simulink model "Exp_300_MPCLinearization"  (R2016a)
settings: Solver=ode45  StartTime=0.0  StopTime=700  RelTol=1e-3
StartFcn:
  | clear all
libraries: mpclib x1
settings Model: Creator=johnh  LastModifiedBy=tiago
settings DataIOCC: SaveFormat=StructureWithTime
settings HardwareCC: ProdWordSize=32  ProdHWDeviceType=Specified
settings ConfigComp: CovModelRefEnable=Off

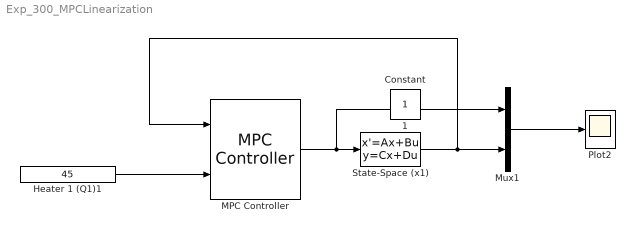
== system Exp_300_MPCLinearization ==
  Heater 1 (Q1)1 : Constant  Value=45
  MPC Controller : mpclib/MPC Controller  SCDEnableBlockLinearizationSpecification=on  mpcobj=mpc1  is_multiple=0  enable_value=0  return_u0=off  ref_from_ws=off  ref_signal_name=[]  ref_preview=off  md_from_ws=off  md_signal_name=[]  md_preview=off  from_project=off  project_file=MPCtask.mat  md_inport=off  mv_inport=off  cost_outport=off  return_sequence=off  return_qpstatus=off  return_state=off  state_inport=off  lims_inport=off  ywt_inport=off  is_designfromscratch=0  uwt_inport=off  duwt_inport=off  rhoeps_inport=off  uref_inport=off  n_ts=0.5  n_mv=1  n_md=1  n_ud=0  n_mo=1  n_uo=0  BlockDataType=double  SampleTimeInherited=off  switch_inport=off
  Mux1 : Mux  Inputs=2
  Plot2 : Scope
  State-Space (x1) : StateSpace  A=-0.005070611210911  B=1.068970183519867e-05  C=3.695395325035177e+02  D=0  X0=0.004775767159700
  1 : Constant  IOType=siggen
  Constant : Constant  IOType=siggen
  wires:
  Mux1/1 -> Plot2/1
  MPC Controller/1 -> State-Space (x1)/1, Mux1/1
  Heater 1 (Q1)1/1 -> MPC Controller/2
  State-Space (x1)/1 -> Mux1/2, MPC Controller/1
